simulink subsystem "flatness_sub"  (R2022b)
settings: Solver=VariableStepAuto  StartTime=0.0  StopTime=10.0  RelTol=1e-3
libraries: dspsigops x1
settings Model: Creator=gotta  LastModifiedBy=gotta

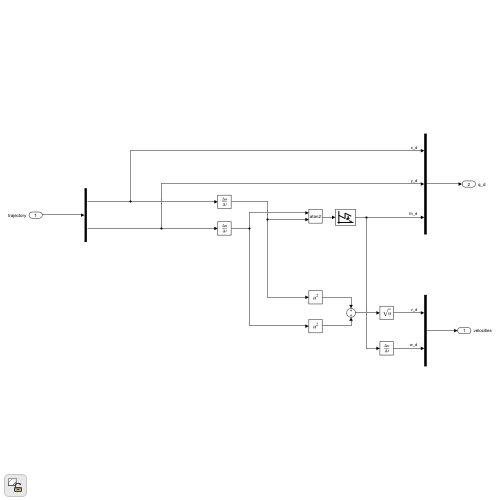
[thumbnail: Simulink's stored preview of the top-level diagram]
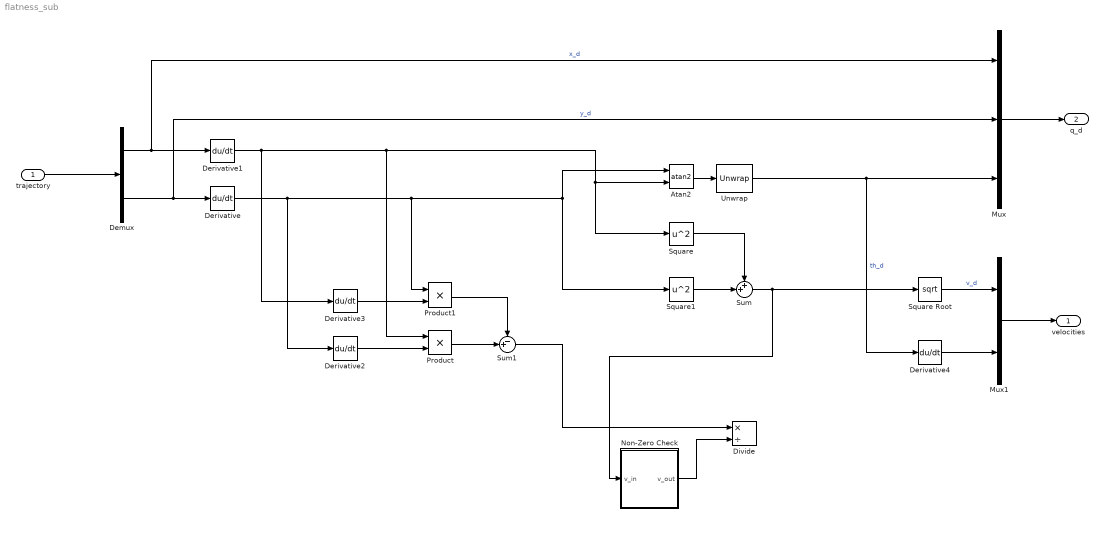
== system flatness_sub ==
  trajectory : Inport
  Atan2 : Trigonometry  Operator=atan2
  Demux : Demux  Outputs=2
  Derivative{,1..4} (5 alike) : Derivative
  Divide : Product  Inputs=*/
  Mux : Mux  Inputs=3
  Mux1 : Mux  Inputs=2
  Non-Zero Check : MATLAB Function  TreatAsAtomicUnit=on
  Product : Product
  Product1 : Product
  Square : Math  Operator=square
  Square Root : Sqrt
  Square1 : Math  Operator=square
  Sum : Sum  Inputs=++|
  Sum1 : Sum  Inputs=-+|
  Unwrap : dspsigops/Unwrap  tol=pi  running=off
  velocities : Outport
  q_d : Outport  Port=2
  wires:
  Sum1/1 -> Divide/1
  Product1/1 -> Sum1/1
  Product/1 -> Sum1/2
  Derivative3/1 -> Product1/2
  Derivative2/1 -> Product/2
  trajectory/1 -> Demux/1
  Unwrap/1 -> Mux/3, Derivative4/1  "th_d"
  Square Root/1 -> Mux1/1  "v_d"
  Mux1/1 -> velocities/1
  Sum/1 -> Square Root/1, Non-Zero Check/1(v_in)
  Square1/1 -> Sum/2
  Square/1 -> Sum/1
  Mux/1 -> q_d/1
  Demux/1 -> Derivative1/1, Mux/1  "x_d"
  Atan2/1 -> Unwrap/1
  Derivative1/1 -> Atan2/2, Square/1, Product/1, Derivative3/1
  Demux/2 -> Derivative/1, Mux/2  "y_d"
  Derivative/1 -> Square1/1, Atan2/1, Product1/1, Derivative2/1
  Non-Zero Check/1(v_out) -> Divide/2
  Derivative4/1 -> Mux1/2

== matlab function flatness_sub/Non-Zero Check ==
  data: v_in input; v_out output
function v_out = fcn(v_in)

if abs(v_in) < 1e-4
    if v_in >= 0 
        v_out = 1e-4;
    else 
        v_out = -1e-4;
    end
else
    v_out = v_in;
end
